simulink model "DOF1_Inverted_Pendulum_Simulation"  (R2020b)
settings: Solver=VariableStepAuto  StartTime=0.0  StopTime=T_sim  RelTol=1e-3
values from neighbouring files (symbols this model uses):
  a = 5.82    [DOF1_Inverted_Pendulum_Params.m]    (also in DOF2_Simulation.m = 0.00368; LQR_Calc_DOF2.m = m_B * l)
  d = 0.001    [DOF1_Inverted_Pendulum_Params.m]
  g = 9.81    [DOF1_Inverted_Pendulum_Params.m]    (also in DOF2_Simulation.m)
  igb = 30    [DOF1_Inverted_Pendulum_Params.m]
  init_theta = 1.00*pi/180    (= 0.0174532925199)    [DOF1_Inverted_Pendulum_Params.m]
  J = 2.175 * 10^-4    (= 0.0002175)    [DOF1_Inverted_Pendulum_Params.m]    (also in DOF2_Simulation.m = 0.000192)
  K = k_m    (= 0.00072032)    [DOF1_Inverted_Pendulum_Params.m]    (also in DOF2_Simulation.m = LQR_Calc_DOF2(K_m,R_m,i_gb,r,m_B,m_W,J,I_2,g,l); LQR_Calc_DOF2.m = lqr(A, B, Q, R))
  Kd = 1.06+ 0    (= 1.06)    [DOF1_Inverted_Pendulum_Params.m]
  Ki = 0   + 0.5    (= 0.5)    [DOF1_Inverted_Pendulum_Params.m]
  Kp = 10  + 2    (= 12)    [DOF1_Inverted_Pendulum_Params.m]
  l = 0.01    [DOF1_Inverted_Pendulum_Params.m]    (also in DOF2_Simulation.m)
  m = 0.368    [DOF1_Inverted_Pendulum_Params.m]
  R = (6.1298+6.7397)/2    (= 6.43475)    [DOF1_Inverted_Pendulum_Params.m]    (also in LQR_Calc_DOF2.m = 0.01)
  tau = 0.016766357422118    (= 0.0167663574221)    [DOF1_Inverted_Pendulum_Params.m]
  yref = 0.00    (= 0)    [DOF1_Inverted_Pendulum_Params.m]
settings Model: Creator=P1_Lenovo  LastModifiedBy=nithi

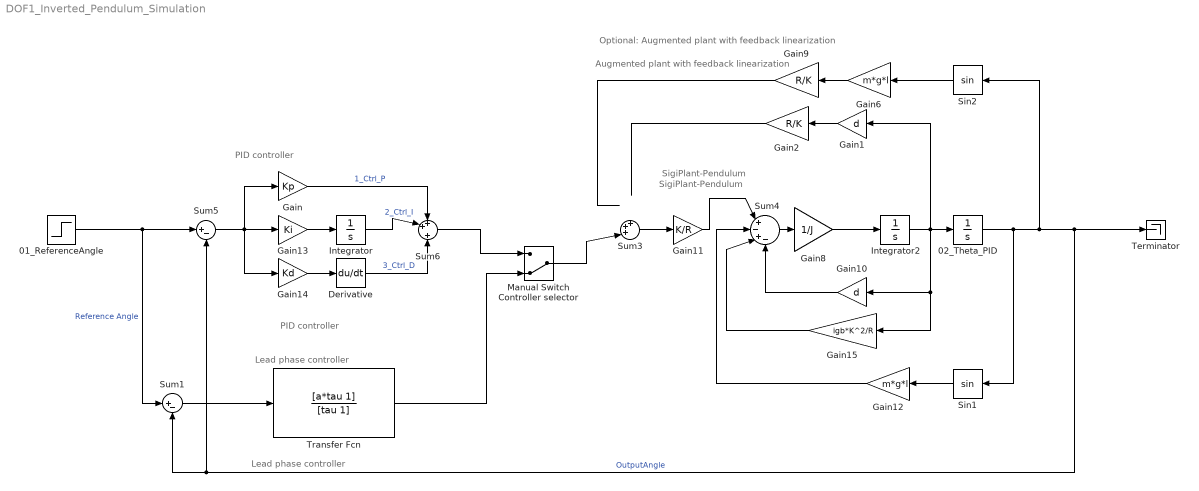
== system DOF1_Inverted_Pendulum_Simulation ==
  note: Lead phase controller
  note: Optional: Augmented plant with feedback linearization
  note: PID controller
  note: Augmented plant with feedback linearization
  note: SigiPlant-Pendulum
  note: PID controller
  note: SigiPlant-Pendulum
  note: Lead phase controller
  01_ReferenceAngle : Step  Time=0  After=yref*1  SampleTime=0
  02_Theta_PID : Integrator  InitialCondition=init_theta*1
  Derivative : Derivative
  Gain : Gain  Gain=Kp
  Gain1 : Gain  Gain=d
  Gain10 : Gain  Gain=d
  Gain11 : Gain  Gain=K/R
  Gain12 : Gain  Gain=m*g*l
  Gain13 : Gain  Gain=Ki
  Gain14 : Gain  Gain=Kd
  Gain15 : Gain  Gain=igb*K^2/R
  Gain2 : Gain  Gain=R/K
  Gain6 : Gain  Gain=m*g*l
  Gain8 : Gain  Gain=1/J
  Gain9 : Gain  Gain=R/K
  Integrator : Integrator
  Integrator2 : Integrator
  Manual Switch Controller selector : ManualSwitch  CurrentSetting=0
  Sin1 : Trigonometry
  Sin2 : Trigonometry
  Sum1 : Sum  Inputs=|+-
  Sum3 : Sum  Inputs=+++|
  Sum4 : Sum  Inputs=|+-+-
  Sum5 : Sum  Inputs=|+-
  Sum6 : Sum  Inputs=++|+
  Terminator : Terminator
  Transfer Fcn : TransferFcn  Numerator=[a*tau 1]  Denominator=[tau 1]
  wires:
  01_ReferenceAngle/1 -> Sum1/1, Sum5/1  "Reference Angle"
  Sum3/1 -> Gain11/1
  Gain9/1 -> ?
  Gain6/1 -> Gain9/1
  Gain11/1 -> Sum4/1
  Gain12/1 -> Sum4/2
  Gain10/1 -> Sum4/4
  Sum4/1 -> Gain8/1
  02_Theta_PID/1 -> Terminator/1, Sum1/2, Sum5/2, Sin2/1, Sin1/1  "OutputAngle"
  Gain8/1 -> Integrator2/1
  Integrator2/1 -> Gain1/1, 02_Theta_PID/1, Gain15/1, Gain10/1
  Sin1/1 -> Gain12/1
  Gain14/1 -> Derivative/1
  Gain13/1 -> Integrator/1
  Derivative/1 -> Sum6/3  "3_Ctrl_D"
  Gain/1 -> Sum6/1  "1_Ctrl_P"
  Integrator/1 -> Sum6/2  "2_Ctrl_I"
  Sum5/1 -> Gain14/1, Gain/1, Gain13/1
  Gain15/1 -> Sum4/3
  Sin2/1 -> Gain6/1
  Gain1/1 -> Gain2/1
  Gain2/1 -> ?
  Sum1/1 -> Transfer Fcn/1
  Sum6/1 -> Manual Switch Controller selector/1
  Transfer Fcn/1 -> Manual Switch Controller selector/2
  Manual Switch Controller selector/1 -> Sum3/3
